simulink model "s2dot2_mux"  (R2023b)
settings: Solver=VariableStepAuto  StartTime=0.0  StopTime=10  RelTol=1e-3
settings Model: Creator=lxj  LastModifiedBy=lxj

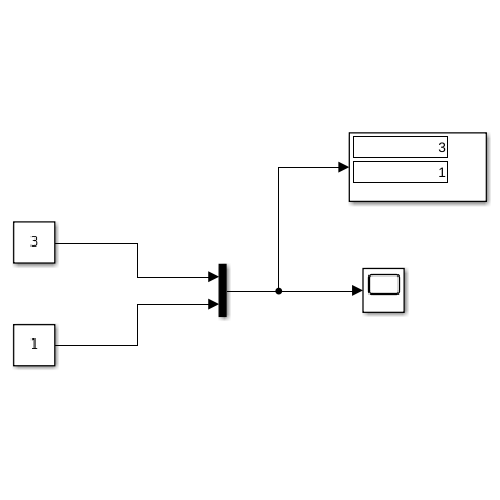
[thumbnail: Simulink's stored preview of the top-level diagram]
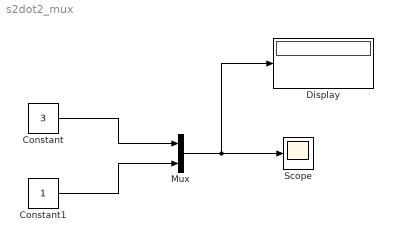
== system s2dot2_mux ==
  Constant : Constant  Value=3
  Constant1 : Constant
  Display : Display
  Mux : Mux  Inputs=2
  Scope : Scope
  wires:
  Constant/1 -> Mux/1
  Constant1/1 -> Mux/2
  Mux/1 -> Display/1, Scope/1
